simulink model "trafo_uc_degistirici"  (R2018a)
settings: Solver=VariableStepAuto  StartTime=0.0  StopTime=1  RelTol=1e-3
libraries: powerlib x17, powerlib_meascontrol x10
settings Model: Creator=ozie  LastModifiedBy=ozie

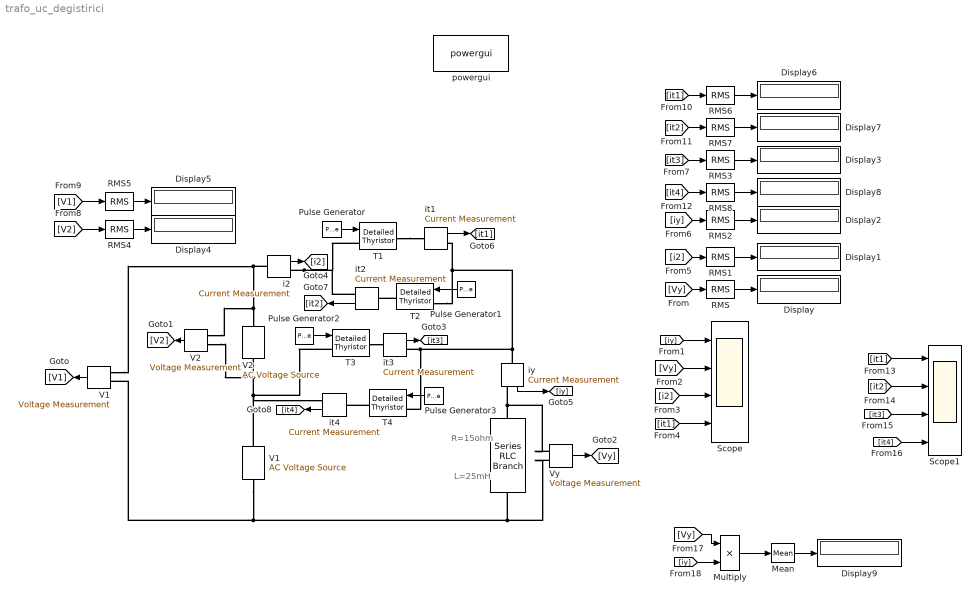
== system trafo_uc_degistirici ==
  note: L=25mH
  note: R=15ohm
  " " : powerlib/Elements/Series RLC Branch  LConnTagsString=__new0  RConnTagsString=__new0  BranchType=RL  Resistance=15  Inductance=25e-3  SetiL0=off  InitialCurrent=0  Capacitance=1e-6  Setx0=off  InitialVoltage=0  Measurements=None
  Display{,1..9} (10 alike) : Display
  Mean : powerlib_meascontrol/Measurements/Mean  Freq=50  Vinit=0  Ts=0
  Multiply : Product
  Pulse Generator : DiscretePulseGenerator  PulseType=Time based  Period=1/50  PulseWidth=5  PhaseDelay=0.01*(90/180)
  Pulse Generator1 : DiscretePulseGenerator  PulseType=Time based  Period=1/50  PulseWidth=5  PhaseDelay=0.01*(270/180)
  Pulse Generator2 : DiscretePulseGenerator  PulseType=Time based  Period=1/50  PulseWidth=5  PhaseDelay=0.01*(0/180)
  Pulse Generator3 : DiscretePulseGenerator  PulseType=Time based  Period=1/50  PulseWidth=5  PhaseDelay=0.01*(180/180)
  RMS{,1..8} (9 alike) : powerlib_meascontrol/Measurements/RMS  TrueRMS=on  Freq=50  RMSInit=120  Ts=0
  Scope : Scope  NumInputPorts=4
  Scope1 : Scope  NumInputPorts=4
  T1 : powerlib/Power Electronics/Detailed Thyristor  Ron=0.001  Lon=1e-3  Vf=0.0001  IL=0.1  Tq=100e-6  IC=0  Rs=1e5  Cs=250e-9  Measurements=off
      settings: SourceProductName=Simscape Power Systems  SourceProductBaseCode=PS
  T2 : powerlib/Power Electronics/Detailed Thyristor  Ron=0.001  Lon=1e-3  Vf=0.0001  IL=0.1  Tq=100e-6  IC=0  Rs=1e5  Cs=250e-9  Measurements=off
      settings: SourceProductName=Simscape Power Systems  SourceProductBaseCode=PS
  "T3 " : powerlib/Power Electronics/Detailed Thyristor  Ron=0.001  Lon=1e-3  Vf=0.0001  IL=0.1  Tq=100e-6  IC=0  Rs=1e5  Cs=250e-9  Measurements=off
      settings: SourceProductName=Simscape Power Systems  SourceProductBaseCode=PS
  T4 : powerlib/Power Electronics/Detailed Thyristor  Ron=0.001  Lon=1e-3  Vf=0.0001  IL=0.1  Tq=100e-6  IC=0  Rs=1e5  Cs=250e-9  Measurements=off
      settings: SourceProductName=Simscape Power Systems  SourceProductBaseCode=PS
  V1 : powerlib/Electrical Sources/AC Voltage Source  Amplitude=220*sqrt(2)  Phase=0  Frequency=50  SampleTime=0  Measurements=None  BusType=swing  Pref=10e3  Qref=0  Qmin=-inf  Qmax=+inf
  "V1  " : powerlib/Measurements/Voltage Measurement  PhasorSimulation=off  OutputType=Complex  PSBequivalent=0
  V2 : powerlib/Electrical Sources/AC Voltage Source  Amplitude=220*sqrt(2)  Phase=0  Frequency=50  SampleTime=0  Measurements=None  BusType=swing  Pref=10e3  Qref=0  Qmin=-inf  Qmax=+inf
  "V2  " : powerlib/Measurements/Voltage Measurement  PhasorSimulation=off  OutputType=Complex  PSBequivalent=0
  Vy : powerlib/Measurements/Voltage Measurement  PhasorSimulation=off  OutputType=Complex  PSBequivalent=0
  i2 : powerlib/Measurements/Current Measurement  PhasorSimulation=off  OutputType=Complex  PSBequivalent=0
  it{1..4} (4 alike) : powerlib/Measurements/Current Measurement  PhasorSimulation=off  OutputType=Complex  PSBequivalent=0
  iy : powerlib/Measurements/Current Measurement  PhasorSimulation=off  OutputType=Complex  PSBequivalent=0
  powergui : powerlib/powergui  Priority=1  SimulationMode=Continuous  SampleTime=50e-6  frequency=60  Iterations=50  frequencyindice=50  Pbase=100e6  ErrMax=1e-4  UnitsV=kV  UnitsW=MW  buscounter=0  FunctionMessages=off  echomessages=off  EnableUseOfTLC=off  CurrentSourceSwitches=off  DisableSnubberDevices=off  DisableRonSwitches=off  DisableVfSwitches=off  DisplayEquations=off  SolverType=Tustin/Backward Euler (TBE)  Interpol=off  ExternalGateDelay=off  methode=off  Ts=100  x0status=blocks  SPID=on  SwTol=0  HookPort=off  RestoreLinks=warning  ResistiveCurrentMeasurement=off  Frange=[0:2:500]  Ylog=off  Xlog=on  ShowGrid=off  save=off  variable=ZData  structure=0  ZoomFFT=off  StartTime=0.0  cycles=1  DisplayStyle=1  fundamental=60  FreqAxis=off  MaxFrequency=1000  frequencyindicesteady=1  RmsSteady=1  display=off
  wires:
  Pulse Generator/1 -> T1/1
  Pulse Generator1/1 -> T2/1
  Pulse Generator2/1 -> "T3 "/1
  Pulse Generator3/1 -> T4/1
  "V1  "/1 -> [V1]
  "V2  "/1 -> [V2]
  Vy/1 -> [Vy]
  i2/1 -> [i2]
  iy/1 -> [iy]
  RMS/1 -> Display/1
  [Vy] -> RMS/1
  [iy] -> Scope/1
  [Vy] -> Scope/2
  [i2] -> Scope/3
  [it1] -> Scope/4
  RMS1/1 -> Display1/1
  [i2] -> RMS1/1
  RMS2/1 -> Display2/1
  [iy] -> RMS2/1
  RMS4/1 -> Display4/1
  [V2] -> RMS4/1
  RMS5/1 -> Display5/1
  [V1] -> RMS5/1
  it1/1 -> [it1]
  RMS6/1 -> Display6/1
  [it1] -> RMS6/1
  it2/1 -> [it2]
  it3/1 -> [it3]
  it4/1 -> [it4]
  RMS7/1 -> Display7/1
  [it2] -> RMS7/1
  RMS8/1 -> Display8/1
  RMS3/1 -> Display3/1
  [it3] -> RMS3/1
  [it4] -> RMS8/1
  [it1] -> Scope1/1
  [it2] -> Scope1/2
  [it3] -> Scope1/3
  [it4] -> Scope1/4
  Mean/1 -> Display9/1
  Multiply/1 -> Mean/1
  [Vy] -> Multiply/1
  [iy] -> Multiply/2
  connections:
  T4/RConn1 -- it4/LConn1
  i2/LConn1 -- "V1  "/LConn1 -- "V2  "/LConn1 -- V2/RConn1
  iy/LConn1 -- it3/RConn1 -- T4/LConn1 -- T2/LConn1 -- it1/RConn1
  Vy/LConn2 -- "V1  "/LConn2 -- V1/LConn1 -- " "/RConn1
  i2/RConn1 -- T1/LConn1 -- it2/RConn1
  Vy/LConn1 -- iy/RConn1 -- " "/LConn1
  T1/RConn1 -- it1/LConn1
  T2/RConn1 -- it2/LConn1
  "T3 "/RConn1 -- it3/LConn1
  "V2  "/LConn2 -- V1/RConn1 -- "T3 "/LConn1 -- it4/RConn1 -- V2/LConn1
